simulink model "SRV02_TF1"  (Simulink 7.3)
settings: Solver=ode45  StartTime=0.0  StopTime=10.0  RelTol=1e-3
settings Model: Creator=Sandor  LastModifiedBy=Sandor

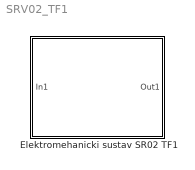
== system SRV02_TF1 ==
  Elektromehanicki sustav SR02 TF1 : Subsystem  mask{Ra=2.6, ke=0.0076776, km=0.007683, Jeq=2e-3, Beq=4e-3, Kg=70, ng=0.9, nm=0.69, w0=0}
      mask prompts: Ra "Otpor armature (Ra)"; ke "Konstanta protuelektromotorne sile (Ke)"; km "Konstanta momenta motora (Km)"; Jeq "Ekvivalentni moment tromosti kod opterecenja (Jeq)"; Beq "Ekvivalentni koeficjent viskoznog trenja Beq"; Kg "SRV02 omjer zupcanika sustava (Kg)"; ng "Korisnost zupcastog prijenosa (Eff_G)"; nm "Korisnost motora (EfF_M)"; w0 "Pocetna kutna brzina(w0)"
      mask help: Nadomjesni model elektromehanickog sustava SR02
      mask Display:
      | port_label('input',1,'Ua')
      | port_label('output',1,'w')

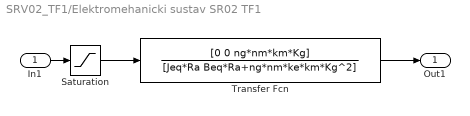
== system SRV02_TF1/Elektromehanicki sustav SR02 TF1 ==
  In1 : Inport
  Saturation : Saturate  UpperLimit=6  LowerLimit=-6  OutDataType=sfix(16)  OutScaling=2^0
  Transfer Fcn : TransferFcn  Numerator=[0 0 ng*nm*km*Kg]  Denominator=[Jeq*Ra Beq*Ra+ng*nm*ke*km*Kg^2]
  Out1 : Outport
  wires:
  In1/1 -> Saturation/1
  Transfer Fcn/1 -> Out1/1
  Saturation/1 -> Transfer Fcn/1
